simulink model "bibli_SM_QUEVAL_20240121_R2021a"  (Simulink 9.3)
settings: Solver=VariableStepAuto  StartTime=0.0  StopTime=10  MaxStep=1e-3  RelTol=1e-3
values from neighbouring files (symbols this model uses):
  Fif = 0.259*3    (= 0.777)    [param_PMSM.m]
  J = 0.5    [param_EESM.m]    (also in param_EESMdampers.m; param_PMSM.m)
  Ld = 1.59e-2    (= 0.0159)    [param_EESM.m]    (also in param_EESMdampers.m; param_PMSM.m)
  Lq = 1.59e-2    (= 0.0159)    [param_EESM.m]    (also in param_EESMdampers.m; param_PMSM.m)
  npp = 2    [param_EESM.m]    (also in param_EESMdampers.m; param_PMSM.m)
undefined symbols (not defined in the file or in its folder): iao_pd_si, ibo_pd_si, ico_pd_si, Ts
undefined symbols (not defined in the file): Clark, fd, InvClark, INVL, M, R
libraries: powerlib x42
(part 1 of 2)
settings Model: Creator=Loïc Queval  LastModifiedBy=Loïc Queval
settings DataIOCC: SaveFormat=Dataset  SignalLoggingSaveFormat=Dataset  ReturnWorkspaceOutputs=on
settings OptimizationCC: LifeSpan=auto
settings DebuggingCC: UnderspecifiedInitializationDetection=Simplified  MergeDetectMultiDrivingBlocksExec=error  FcnCallInpInsideContextMsg=error  UnconnectedInputMsg=none  UnconnectedOutputMsg=none  UnconnectedLineMsg=none  SFUnexpectedBacktrackingDiag=error  SFNoUnconditionalDefaultTransitionDiag=error  SFExecutionAtInitializationDiag=warning  ArithmeticOperatorsInVariantConditions=error
settings HardwareCC: ProdBitPerPointer=64  ProdBitPerSizeT=64  ProdBitPerPtrDiffT=64  ProdLargestAtomicFloat=Float  ProdIntDivRoundTo=Zero  ProdEndianess=LittleEndian  ProdWordSize=64  ProdHWDeviceType=Intel->x86-64 (Windows64)
settings ModelReferenceCC: EnableRefExpFcnMdlSchedulingChecks=off  PropagateSignalLabelsOutOfModel=on
settings SFSimCC: SimUseLocalCustomCode=on
settings RTWCC: RTWUseLocalCustomCode=on
settings CodeAppCC: StateflowObjectComments=off
settings GRTTargetCC: TargetLangStandard=C99 (ISO)  CombineOutputUpdateFcns=on  GRTInterface=off
settings ConfigComp: CovMetricSettings=dwe  CovSaveCumulativeToWorkspaceVar=off  CovSaveSingleToWorkspaceVar=off  CovExternalEMLEnable=on

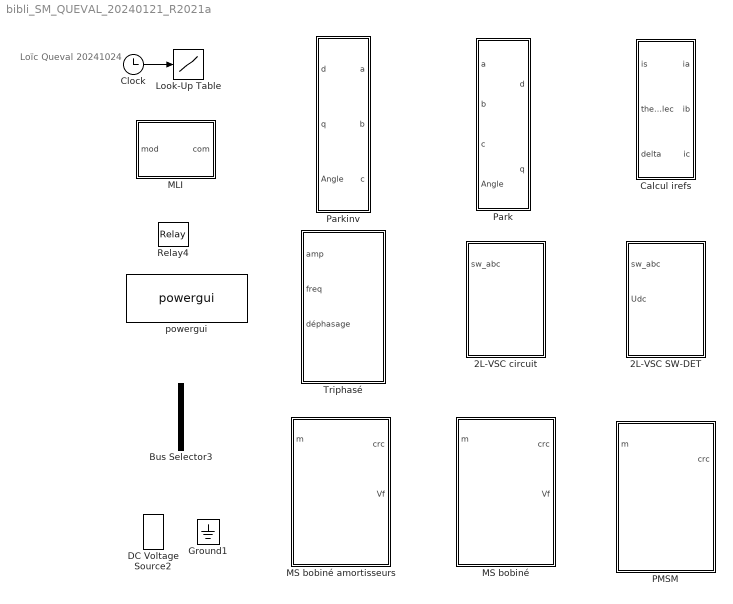
== system bibli_SM_QUEVAL_20240121_R2021a ==
  note: Loïc Queval
      | 20241024
  2L-VSC SW-DET : Subsystem
  2L-VSC circuit : Subsystem
  Bus Selector3 : BusSelector  OutputSignals=Cm,Vit,ia,v_an
  Calcul irefs : Subsystem
  Clock : Clock
  DC Voltage Source2 : powerlib/Electrical Sources/DC Voltage Source  Amplitude=300  Measurements=None
  Ground1 : powerlib/Elements/Ground  LConnTagsString=a
  Look-Up Table : Lookup  InputValues=[0 4 4 6 6 10]  Table=[0 0 30 30 100 100]  SaturateOnIntegerOverflow=on
  MLI : Subsystem
  MS bobiné : Subsystem
  MS bobiné amortisseurs : Subsystem
  PMSM : Subsystem
  Park : Subsystem
  Parkinv : Subsystem
  Relay4 : Relay  OnSwitchValue=1  OffSwitchValue=-1
  Triphasé : Subsystem
  powergui : powerlib/powergui  SimulationMode=Continuous  SampleTime=Ts  frequency=60  Iterations=50  frequencyindice=0  Pbase=100e6  ErrMax=1e-4  UnitsV=kV  UnitsW=MW  buscounter=0  FunctionMessages=off  echomessages=off  EnableUseOfTLC=off  CurrentSourceSwitches=off  DisableSnubberDevices=off  DisableRonSwitches=off  DisableVfSwitches=off  DisplayEquations=off  AutomaticDiscreteSolvers=off  SolverType=Tustin/Backward Euler (TBE)  Interpol=off  ExternalGateDelay=off  methode=off  Ts=0  x0status=blocks  SPID=off  SwTol=0  HookPort=off  NonlinearTolerance=1e-4  nMaxIteration=100  ContinueOnMaxIteration=off  RestoreLinks=warning  ResistiveCurrentMeasurement=off  Frange=[0:2:500]  Ylog=off  Xlog=on  ShowGrid=off  save=off  variable=ZData  structure=data_PWM  ZoomFFT=off  StartTime=0.02  cycles=1  DisplayStyle=1  fundamental=50  FreqAxis=on  MaxFrequency=1000  frequencyindicesteady=1  RmsSteady=1  display=off
  wires:
  Clock/1 -> Look-Up Table/1

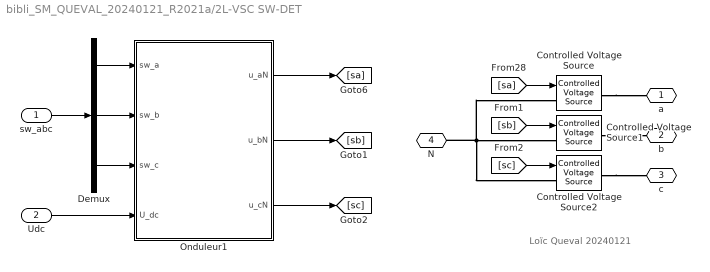
== system bibli_SM_QUEVAL_20240121_R2021a/2L-VSC SW-DET ==
  note: Loïc Queval
      | 20240121
  sw_abc : Inport
  Udc : Inport  Port=2
  Controlled Voltage Source : powerlib/Electrical Sources/Controlled Voltage Source  Initialize=off  Source_Type=AC  Amplitude=0  Phase=0  Frequency=0  Measurements=None
  Controlled Voltage Source1 : powerlib/Electrical Sources/Controlled Voltage Source  Initialize=off  Source_Type=AC  Amplitude=0  Phase=0  Frequency=0  Measurements=None
  Controlled Voltage Source2 : powerlib/Electrical Sources/Controlled Voltage Source  Initialize=off  Source_Type=AC  Amplitude=0  Phase=0  Frequency=0  Measurements=None
  Demux : Demux  Outputs=3
  Onduleur1 : Subsystem
  a : PMIOPort  Side=Right
  b : PMIOPort  Port=2  Side=Right
  c : PMIOPort  Port=3  Side=Right
  N : PMIOPort  Port=4  Side=Left
  wires:
  Demux/1 -> Onduleur1/1(sw_a)
  [sa] -> Controlled Voltage Source/1
  [sb] -> Controlled Voltage Source1/1
  [sc] -> Controlled Voltage Source2/1
  Demux/2 -> Onduleur1/2(sw_b)
  Demux/3 -> Onduleur1/3(sw_c)
  Udc/1 -> Onduleur1/4(U_dc)
  Onduleur1/3(u_cN) -> [sc]
  Onduleur1/1(u_aN) -> [sa]
  Onduleur1/2(u_bN) -> [sb]
  sw_abc/1 -> Demux/1
  connections:
  Controlled Voltage Source/RConn1 -- a/RConn1
  Controlled Voltage Source1/RConn1 -- b/RConn1
  Controlled Voltage Source2/RConn1 -- c/RConn1
  N/RConn1 -- Controlled Voltage Source2/LConn1 -- Controlled Voltage Source1/LConn1 -- Controlled Voltage Source/LConn1

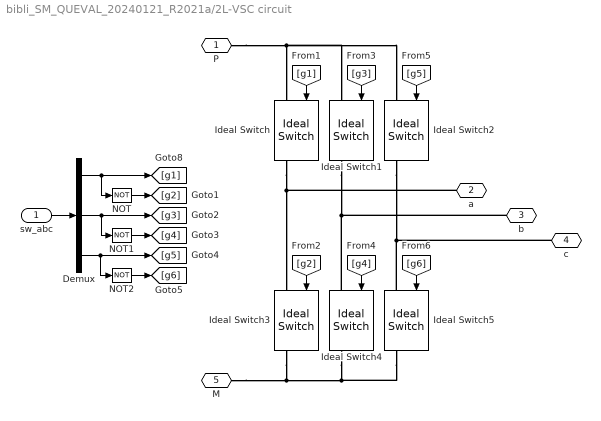
== system bibli_SM_QUEVAL_20240121_R2021a/2L-VSC circuit ==
  sw_abc : Inport
  Demux : Demux  Outputs=3
  Ideal Switch{,1..5} (6 alike) : powerlib/Power Electronics/Ideal Switch  Ron=0.001  Lon=0  IC=0  Rs=1e5  Cs=inf  Measurements=on
  NOT : Logic  Operator=NOT  IconShape=distinctive  AllPortsSameDT=off  OutDataTypeStr=boolean
  NOT1 : Logic  Operator=NOT  IconShape=distinctive  AllPortsSameDT=off  OutDataTypeStr=boolean
  NOT2 : Logic  Operator=NOT  IconShape=distinctive  AllPortsSameDT=off  OutDataTypeStr=boolean
  P : PMIOPort  Side=Left
  a : PMIOPort  Port=2  Side=Right
  b : PMIOPort  Port=3  Side=Right
  c : PMIOPort  Port=4  Side=Right
  M : PMIOPort  Port=5  Side=Left
  wires:
  sw_abc/1 -> Demux/1
  [g1] -> Ideal Switch/1
  [g2] -> Ideal Switch3/1
  [g3] -> Ideal Switch1/1
  [g4] -> Ideal Switch4/1
  [g5] -> Ideal Switch2/1
  [g6] -> Ideal Switch5/1
  NOT1/1 -> [g4]
  Demux/1 -> NOT/1, [g1]
  NOT/1 -> [g2]
  NOT2/1 -> [g6]
  Demux/2 -> NOT1/1, [g3]
  Demux/3 -> NOT2/1, [g5]
  connections:
  b/RConn1 -- Ideal Switch4/LConn1 -- Ideal Switch1/RConn1
  a/RConn1 -- Ideal Switch/RConn1 -- Ideal Switch3/LConn1
  M/RConn1 -- Ideal Switch3/RConn1 -- Ideal Switch5/RConn1 -- Ideal Switch4/RConn1
  P/RConn1 -- Ideal Switch2/LConn1 -- Ideal Switch1/LConn1 -- Ideal Switch/LConn1
  c/RConn1 -- Ideal Switch5/LConn1 -- Ideal Switch2/RConn1

== system bibli_SM_QUEVAL_20240121_R2021a/Calcul irefs ==
  is : Inport
  thetelec : Inport  Port=2
  delta : Inport  Port=3
  Fcn : Fcn  Expr=u[1]*cos(u[2]+u[3])
  Fcn1 : Fcn  Expr=u[1]*cos(u[2]-2*pi/3+u[3])
  Fcn2 : Fcn  Expr=u[1]*cos(u[2]-4*pi/3+u[3])
  Mux : Mux  Inputs=3
  ia : Outport  InitialOutput=0  VectorParamsAs1DForOutWhenUnconnected=off
  ib : Outport  Port=2  InitialOutput=0  VectorParamsAs1DForOutWhenUnconnected=off
  ic : Outport  Port=3  InitialOutput=0  VectorParamsAs1DForOutWhenUnconnected=off
  wires:
  Mux/1 -> Fcn1/1, Fcn2/1, Fcn/1
  Fcn/1 -> ia/1
  is/1 -> Mux/1
  Fcn1/1 -> ib/1
  thetelec/1 -> Mux/2
  Fcn2/1 -> ic/1
  delta/1 -> Mux/3

== system bibli_SM_QUEVAL_20240121_R2021a/MLI ==
  note: Définir la fréquence de découpage fd
  mod : Inport
  Relay : Relay  OnSwitchValue=0  OffSwitchValue=0
  Repeating Sequence : Subsystem  mask(Repeating table){Parameter1=[0 0.25/fd 0.75/fd 1/fd], Parameter2=[0 1 -1 0]}
      mask prompts: Parameter1 "Time values:"; Parameter2 "Output values:"
      mask help:
      | Repeating table.
      | Enter values of time and output for first cycle.
      mask init:
      | period = max(@1); t = @1; y = @2;
      mask Help: Repeats cycle given in table. Time values should be monotonically increasing.
      mask Display: plot([t,t+period,t+2*period],[y,y,y])
  Sum : Sum  Inputs=+-  InputSameDT=on  SaturateOnIntegerOverflow=on  OutDataTypeStr=Inherit: Same as first input
  com : Outport  VectorParamsAs1DForOutWhenUnconnected=off
  wires:
  Repeating Sequence/1(out_1) -> Sum/2
  Sum/1 -> Relay/1
  mod/1 -> Sum/1
  Relay/1 -> com/1

== system bibli_SM_QUEVAL_20240121_R2021a/MS bobiné ==
  note: ELECTRICAL TERMINATORS
      | OF THE MACHINE
  note: <----- ia
  note: Loïc Queval
      | 20240109
  note: current must go out!
  crc : Inport
  Vf : Inport  Port=2
  CURRENT INJECTION SYSTEM Converts Simulink signals into currents : Subsystem
  Gain : Gain  Gain=-1
  MS bobiné : Subsystem
  VOLTAGE MEASUREMENT SYSTEM Converts voltages into  Simulink signals : Subsystem
  n : PMIOPort  Side=Left
  a : PMIOPort  Port=2  Side=Right
  b : PMIOPort  Port=3  Side=Right
  c : PMIOPort  Port=4  Side=Right
  m : Outport
  wires:
  VOLTAGE MEASUREMENT SYSTEM Converts voltages into  Simulink signals/1(voltages) -> MS bobiné/1(voltages)
  MS bobiné/1(currents) -> Gain/1
  MS bobiné/2(m) -> m/1
  Gain/1 -> CURRENT INJECTION SYSTEM Converts Simulink signals into currents/1(currents)
  Vf/1 -> MS bobiné/3(Vf)
  crc/1 -> MS bobiné/2(crc)
  connections:
  a/RConn1 -- CURRENT INJECTION SYSTEM Converts Simulink signals into currents/RConn1 -- VOLTAGE MEASUREMENT SYSTEM Converts voltages into  Simulink signals/LConn1
  VOLTAGE MEASUREMENT SYSTEM Converts voltages into  Simulink signals/LConn2 -- CURRENT INJECTION SYSTEM Converts Simulink signals into currents/RConn2 -- b/RConn1
  VOLTAGE MEASUREMENT SYSTEM Converts voltages into  Simulink signals/LConn3 -- CURRENT INJECTION SYSTEM Converts Simulink signals into currents/RConn3 -- c/RConn1
  n/RConn1 -- CURRENT INJECTION SYSTEM Converts Simulink signals into currents/RConn4 -- VOLTAGE MEASUREMENT SYSTEM Converts voltages into  Simulink signals/LConn4

== system bibli_SM_QUEVAL_20240121_R2021a/MS bobiné amortisseurs ==
  note: ELECTRICAL TERMINATORS
      | OF THE MACHINE
  note: <----- ia
  note: Loïc Queval
      | 20240109
  note: current must go out!
  crc : Inport
  Vf : Inport  Port=2
  CURRENT INJECTION SYSTEM Converts Simulink signals into currents : Subsystem
  Gain : Gain  Gain=-1
  MS bobiné amortisseurs : Subsystem
  VOLTAGE MEASUREMENT SYSTEM Converts voltages into  Simulink signals : Subsystem
  n : PMIOPort  Side=Left
  a : PMIOPort  Port=2  Side=Right
  b : PMIOPort  Port=3  Side=Right
  c : PMIOPort  Port=4  Side=Right
  m : Outport
  wires:
  VOLTAGE MEASUREMENT SYSTEM Converts voltages into  Simulink signals/1(voltages) -> MS bobiné amortisseurs/1(voltages)
  MS bobiné amortisseurs/1(currents) -> Gain/1
  MS bobiné amortisseurs/2(m) -> m/1
  Gain/1 -> CURRENT INJECTION SYSTEM Converts Simulink signals into currents/1(currents)
  crc/1 -> MS bobiné amortisseurs/2(crc)
  Vf/1 -> MS bobiné amortisseurs/3(Vf)
  connections:
  a/RConn1 -- CURRENT INJECTION SYSTEM Converts Simulink signals into currents/RConn1 -- VOLTAGE MEASUREMENT SYSTEM Converts voltages into  Simulink signals/LConn1
  VOLTAGE MEASUREMENT SYSTEM Converts voltages into  Simulink signals/LConn2 -- CURRENT INJECTION SYSTEM Converts Simulink signals into currents/RConn2 -- b/RConn1
  VOLTAGE MEASUREMENT SYSTEM Converts voltages into  Simulink signals/LConn3 -- CURRENT INJECTION SYSTEM Converts Simulink signals into currents/RConn3 -- c/RConn1
  n/RConn1 -- CURRENT INJECTION SYSTEM Converts Simulink signals into currents/RConn4 -- VOLTAGE MEASUREMENT SYSTEM Converts voltages into  Simulink signals/LConn4

== system bibli_SM_QUEVAL_20240121_R2021a/PMSM ==
  note: ELECTRICAL TERMINATORS
      | OF THE MACHINE
  note: <----- ia
  note: Loïc Queval
      | 20240120
  note: current must go out!
  crc : Inport
  CURRENT INJECTION SYSTEM Converts Simulink signals into currents : Subsystem
  Gain : Gain  Gain=-1
  PMSM : Subsystem
  VOLTAGE MEASUREMENT SYSTEM Converts voltages into  Simulink signals : Subsystem
  n : PMIOPort  Side=Left
  a : PMIOPort  Port=2  Side=Right
  b : PMIOPort  Port=3  Side=Right
  c : PMIOPort  Port=4  Side=Right
  m : Outport
  wires:
  VOLTAGE MEASUREMENT SYSTEM Converts voltages into  Simulink signals/1(voltages) -> PMSM/1(voltages)
  PMSM/1(currents) -> Gain/1
  PMSM/2(m) -> m/1
  Gain/1 -> CURRENT INJECTION SYSTEM Converts Simulink signals into currents/1(currents)
  crc/1 -> PMSM/2(crc)
  connections:
  CURRENT INJECTION SYSTEM Converts Simulink signals into currents/RConn1 -- a/RConn1 -- VOLTAGE MEASUREMENT SYSTEM Converts voltages into  Simulink signals/LConn1
  CURRENT INJECTION SYSTEM Converts Simulink signals into currents/RConn2 -- VOLTAGE MEASUREMENT SYSTEM Converts voltages into  Simulink signals/LConn2 -- b/RConn1
  VOLTAGE MEASUREMENT SYSTEM Converts voltages into  Simulink signals/LConn3 -- c/RConn1 -- CURRENT INJECTION SYSTEM Converts Simulink signals into currents/RConn3
  n/RConn1 -- CURRENT INJECTION SYSTEM Converts Simulink signals into currents/RConn4 -- VOLTAGE MEASUREMENT SYSTEM Converts voltages into  Simulink signals/LConn4

== system bibli_SM_QUEVAL_20240121_R2021a/Park ==
  a : Inport
  b : Inport  Port=2
  c : Inport  Port=3
  Angle : Inport  Port=4
  Clark : Subsystem
  Rotation : Subsystem
  Trigonometric Function : Trigonometry
  Trigonometric Function1 : Trigonometry  Operator=cos
  d : Outport  InitialOutput=0  VectorParamsAs1DForOutWhenUnconnected=off
  q : Outport  Port=2  InitialOutput=0  VectorParamsAs1DForOutWhenUnconnected=off
  wires:
  Rotation/1(d) -> d/1
  Rotation/2(q) -> q/1
  b/1 -> Clark/2(b)
  c/1 -> Clark/3(c)
  a/1 -> Clark/1(a)
  Clark/1(alpha) -> Rotation/3(alpha)
  Clark/2(beta) -> Rotation/4(beta)
  Trigonometric Function/1 -> Rotation/2(sin)
  Trigonometric Function1/1 -> Rotation/1(cos)
  Angle/1 -> Trigonometric Function1/1, Trigonometric Function/1

== system bibli_SM_QUEVAL_20240121_R2021a/Parkinv ==
  d : Inport
  q : Inport  Port=2
  Angle : Inport  Port=3
  ClarkInv : Subsystem
  Rotation Inverse : Subsystem
  Trigonometric Function : Trigonometry
  Trigonometric Function1 : Trigonometry  Operator=cos
  a : Outport  InitialOutput=0  VectorParamsAs1DForOutWhenUnconnected=off
  b : Outport  Port=2  InitialOutput=0  VectorParamsAs1DForOutWhenUnconnected=off
  c : Outport  Port=3  InitialOutput=0  VectorParamsAs1DForOutWhenUnconnected=off
  wires:
  Rotation Inverse/1(alpha) -> ClarkInv/1(alpha)
  ClarkInv/1(a) -> a/1
  ClarkInv/2(b) -> b/1
  d/1 -> Rotation Inverse/3(d)
  ClarkInv/3(c) -> c/1
  q/1 -> Rotation Inverse/4(q)
  Rotation Inverse/2(beta) -> ClarkInv/2(beta)
  Trigonometric Function/1 -> Rotation Inverse/2(sin)
  Trigonometric Function1/1 -> Rotation Inverse/1(cos)
  Angle/1 -> Trigonometric Function1/1, Trigonometric Function/1

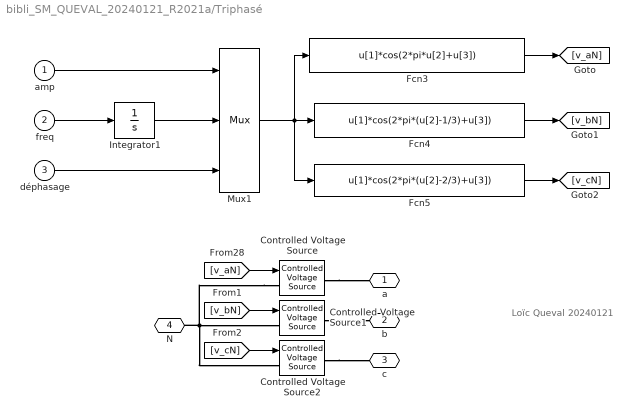
== system bibli_SM_QUEVAL_20240121_R2021a/Triphasé ==
  note: Loïc Queval
      | 20240121
  amp : Inport
  freq : Inport  Port=2
  déphasage : Inport  Port=3
  Controlled Voltage Source : powerlib/Electrical Sources/Controlled Voltage Source  Initialize=on  Source_Type=AC  Amplitude=0  Phase=0  Frequency=0  Measurements=None
  Controlled Voltage Source1 : powerlib/Electrical Sources/Controlled Voltage Source  Initialize=on  Source_Type=AC  Amplitude=0  Phase=0  Frequency=0  Measurements=None
  Controlled Voltage Source2 : powerlib/Electrical Sources/Controlled Voltage Source  Initialize=on  Source_Type=AC  Amplitude=0  Phase=0  Frequency=0  Measurements=None
  Fcn3 : Fcn  Expr=u[1]*cos(2*pi*u[2]+u[3])
  Fcn4 : Fcn  Expr=u[1]*cos(2*pi*(u[2]-1/3)+u[3])
  Fcn5 : Fcn  Expr=u[1]*cos(2*pi*(u[2]-2/3)+u[3])
  Integrator1 : Integrator
  Mux1 : Mux  Inputs=3
  a : PMIOPort  Side=Right
  b : PMIOPort  Port=2  Side=Right
  c : PMIOPort  Port=3  Side=Right
  N : PMIOPort  Port=4  Side=Left
  wires:
  Fcn5/1 -> [v_cN]
  Fcn4/1 -> [v_bN]
  Fcn3/1 -> [v_aN]
  [v_aN] -> Controlled Voltage Source/1
  [v_bN] -> Controlled Voltage Source1/1
  [v_cN] -> Controlled Voltage Source2/1
  Integrator1/1 -> Mux1/2
  amp/1 -> Mux1/1
  Mux1/1 -> Fcn4/1, Fcn5/1, Fcn3/1
  freq/1 -> Integrator1/1
  déphasage/1 -> Mux1/3
  connections:
  Controlled Voltage Source/LConn1 -- N/RConn1 -- Controlled Voltage Source2/LConn1 -- Controlled Voltage Source1/LConn1
  Controlled Voltage Source1/RConn1 -- b/RConn1
  Controlled Voltage Source2/RConn1 -- c/RConn1
  Controlled Voltage Source/RConn1 -- a/RConn1

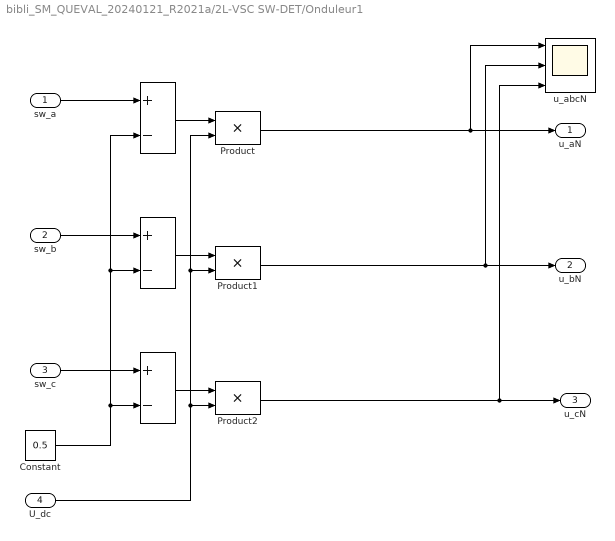
== system bibli_SM_QUEVAL_20240121_R2021a/2L-VSC SW-DET/Onduleur1 ==
  sw_a : Inport
  sw_b : Inport  Port=2
  sw_c : Inport  Port=3
  U_dc : Inport  Port=4
  " " : Sum  Inputs=+-  InputSameDT=on  SaturateOnIntegerOverflow=on  OutDataTypeStr=Inherit: Same as first input
  "  " : Sum  Inputs=+-  InputSameDT=on  SaturateOnIntegerOverflow=on  OutDataTypeStr=Inherit: Same as first input
  "   " : Sum  Inputs=+-  InputSameDT=on  SaturateOnIntegerOverflow=on  OutDataTypeStr=Inherit: Same as first input
  Constant : Constant  Value=0.5
  Product : Product  InputSameDT=on  SaturateOnIntegerOverflow=on  OutDataTypeStr=Inherit: Same as first input
  Product1 : Product  InputSameDT=on  SaturateOnIntegerOverflow=on  OutDataTypeStr=Inherit: Same as first input
  Product2 : Product  InputSameDT=on  SaturateOnIntegerOverflow=on  OutDataTypeStr=Inherit: Same as first input
  u_abcN : Scope  NumInputPorts=3
  u_aN : Outport  VectorParamsAs1DForOutWhenUnconnected=off
  u_bN : Outport  Port=2  VectorParamsAs1DForOutWhenUnconnected=off
  u_cN : Outport  Port=3  VectorParamsAs1DForOutWhenUnconnected=off
  wires:
  sw_a/1 -> " "/1
  sw_b/1 -> "   "/1
  sw_c/1 -> "  "/1
  Product/1 -> u_abcN/1, u_aN/1
  " "/1 -> Product/1
  "   "/1 -> Product1/1
  "  "/1 -> Product2/1
  U_dc/1 -> Product/2, Product1/2, Product2/2
  Constant/1 -> " "/2, "   "/2, "  "/2
  Product1/1 -> u_abcN/2, u_bN/1
  Product2/1 -> u_abcN/3, u_cN/1

== system bibli_SM_QUEVAL_20240121_R2021a/MLI/Repeating Sequence ==
  Clock : Clock
  Fcn1 : Fcn  Expr=rem(u[1],period)
  Look-Up Table : Lookup  InputValues=t  Table=y  SaturateOnIntegerOverflow=on
  out_1 : Outport  InitialOutput=0  VectorParamsAs1DForOutWhenUnconnected=off
  wires:
  Look-Up Table/1 -> out_1/1
  Clock/1 -> Fcn1/1
  Fcn1/1 -> Look-Up Table/1

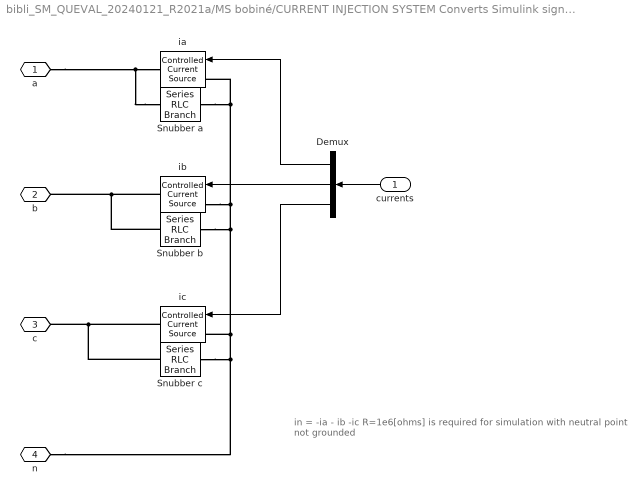
== system bibli_SM_QUEVAL_20240121_R2021a/MS bobiné/CURRENT INJECTION SYSTEM Converts Simulink signals into currents ==
  note: in = -ia - ib -ic
      | R=1e6[ohms] is required for simulation with neutral point not grounded
  currents : Inport
  Demux : Demux  Outputs=3
  Snubber a : powerlib/Elements/Series RLC Branch  LConnTagsString=__new0  RConnTagsString=__new0  BranchType=R  Resistance=1e6  Inductance=1e-3  SetiL0=off  InitialCurrent=0  Capacitance=1e-6  Setx0=off  InitialVoltage=0  Measurements=None
  Snubber b : powerlib/Elements/Series RLC Branch  LConnTagsString=__new0  RConnTagsString=__new0  BranchType=R  Resistance=1e6  Inductance=1e-3  SetiL0=off  InitialCurrent=0  Capacitance=1e-6  Setx0=off  InitialVoltage=0  Measurements=None
  Snubber c : powerlib/Elements/Series RLC Branch  LConnTagsString=__new0  RConnTagsString=__new0  BranchType=R  Resistance=1e6  Inductance=1e-3  SetiL0=off  InitialCurrent=0  Capacitance=1e-6  Setx0=off  InitialVoltage=0  Measurements=None
  ia : powerlib/Electrical Sources/Controlled Current Source  Initialize=off  Source_Type=DC  Amplitude=-iao_pd_si  Phase=0  Frequency=0  Measurements=None
  ib : powerlib/Electrical Sources/Controlled Current Source  Initialize=off  Source_Type=DC  Amplitude=-ibo_pd_si  Phase=0  Frequency=0  Measurements=None
  ic : powerlib/Electrical Sources/Controlled Current Source  Initialize=off  Source_Type=DC  Amplitude=-ico_pd_si  Phase=0  Frequency=0  Measurements=None
  a : PMIOPort  Side=Right
  b : PMIOPort  Port=2  Side=Right
  c : PMIOPort  Port=3  Side=Right
  n : PMIOPort  Port=4  Side=Right
  wires:
  Demux/1 -> ia/1
  Demux/2 -> ib/1
  currents/1 -> Demux/1
  Demux/3 -> ic/1
  connections:
  Snubber a/LConn1 -- a/RConn1 -- ia/RConn1
  ib/RConn1 -- b/RConn1 -- Snubber b/LConn1
  Snubber b/RConn1 -- Snubber a/RConn1 -- ia/LConn1 -- ib/LConn1 -- ic/LConn1 -- Snubber c/RConn1 -- n/RConn1
  Snubber c/LConn1 -- ic/RConn1 -- c/RConn1

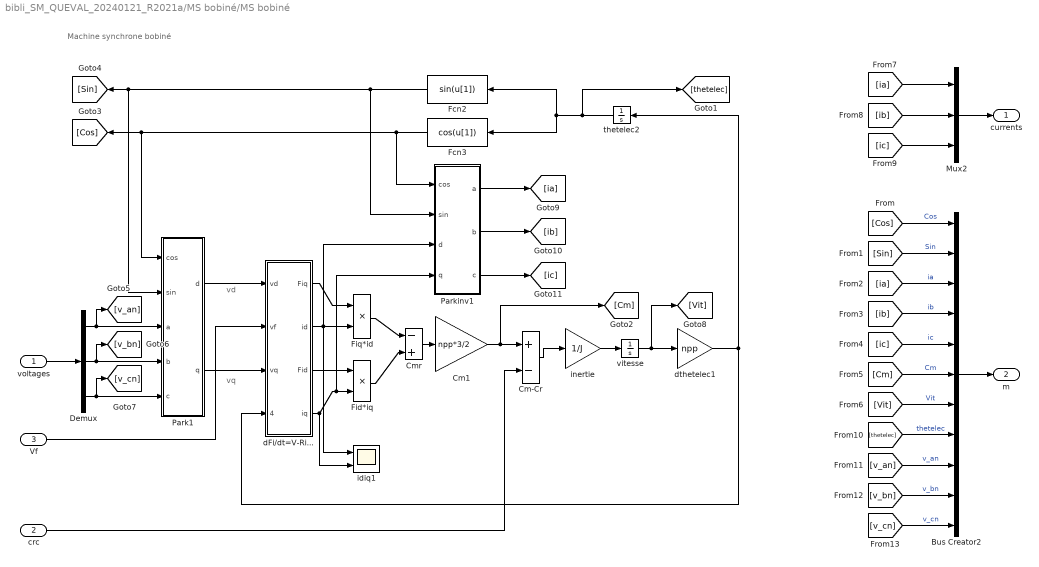
== system bibli_SM_QUEVAL_20240121_R2021a/MS bobiné/MS bobiné ==
  note: Machine synchrone bobiné
  note: vd
  note: vq
  voltages : Inport
  crc : Inport  Port=2
  Vf : Inport  Port=3
  Bus Creator2 : BusCreator  Inputs=11
  Cm-Cr : Sum  Inputs=+-  InputSameDT=on  SaturateOnIntegerOverflow=on  OutDataTypeStr=Inherit: Same as first input
  Cm1 : Gain  Gain=npp*3/2  SaturateOnIntegerOverflow=on  OutDataTypeStr=Inherit: Same as input  ParamDataTypeStr=Inherit: Same as input
  Cmr : Sum  Inputs=-+  InputSameDT=on  SaturateOnIntegerOverflow=on  OutDataTypeStr=Inherit: Same as first input
  Demux : Demux  Outputs=3
  Fcn2 : Fcn
  Fcn3 : Fcn  Expr=cos(u[1])
  "Fid*iq " : Product  InputSameDT=on  RndMeth=Zero  SaturateOnIntegerOverflow=on  OutDataTypeStr=Inherit: Same as first input
  Fiq*id : Product  InputSameDT=on  RndMeth=Zero  SaturateOnIntegerOverflow=on  OutDataTypeStr=Inherit: Same as first input
  Mux2 : Mux  Inputs=3
  Park1 : Subsystem
  Parkinv1 : Subsystem
  dFi/dt=V-Ri... : Subsystem
  dthetelec1 : Gain  Gain=npp  SaturateOnIntegerOverflow=on  OutDataTypeStr=Inherit: Same as input  ParamDataTypeStr=Inherit: Same as input
  idiq1 : Scope  NumInputPorts=2
  inertie : Gain  Gain=1/J  SaturateOnIntegerOverflow=on  OutDataTypeStr=Inherit: Same as input  ParamDataTypeStr=Inherit: Same as input
  thetelec2 : Integrator
  vitesse : Integrator
  currents : Outport
  m : Outport  Port=2
  wires:
  Mux2/1 -> currents/1
  Bus Creator2/1 -> m/1
  [Vit] -> Bus Creator2/7  "Vit"
  [Cm] -> Bus Creator2/6  "Cm"
  [ic] -> Bus Creator2/5  "ic"
  [ib] -> Bus Creator2/4  "ib"
  [ia] -> Bus Creator2/3  "ia"
  [Sin] -> Bus Creator2/2  "Sin"
  [Cos] -> Bus Creator2/1  "Cos"
  [ia] -> Mux2/1
  [ib] -> Mux2/2
  [ic] -> Mux2/3
  [thetelec] -> Bus Creator2/8  "thetelec"
  dFi/dt=V-Ri.../3(Fid) -> "Fid*iq "/1
  "Fid*iq "/1 -> Cmr/2
  Fiq*id/1 -> Cmr/1
  Fcn3/1 -> Parkinv1/1(cos), Park1/1(cos), [Cos]
  dFi/dt=V-Ri.../1(Fiq) -> Fiq*id/1
  Demux/2 -> [v_bn], Park1/4(b)
  Cmr/1 -> Cm1/1
  dFi/dt=V-Ri.../4(iq) -> idiq1/2, Parkinv1/4(q), "Fid*iq "/2
  Park1/1(d) -> dFi/dt=V-Ri.../1(vd)
  dFi/dt=V-Ri.../2(id) -> idiq1/1, Parkinv1/3(d), Fiq*id/2
  Cm-Cr/1 -> inertie/1
  Vf/1 -> dFi/dt=V-Ri.../2(vf)
  vitesse/1 -> [Vit], dthetelec1/1
  Fcn2/1 -> Parkinv1/2(sin), [Sin], Park1/2(sin)
  inertie/1 -> vitesse/1
  thetelec2/1 -> [thetelec], Fcn2/1, Fcn3/1
  Demux/3 -> [v_cn], Park1/5(c)
  Cm1/1 -> [Cm], Cm-Cr/1
  dthetelec1/1 -> thetelec2/1, dFi/dt=V-Ri.../4(dthetelec)
  Parkinv1/1(a) -> [ia]
  Parkinv1/3(c) -> [ic]
  Demux/1 -> [v_an], Park1/3(a)
  Parkinv1/2(b) -> [ib]
  Park1/2(q) -> dFi/dt=V-Ri.../3(vq)
  voltages/1 -> Demux/1
  crc/1 -> Cm-Cr/2
  [v_cn] -> Bus Creator2/11  "v_cn"
  [v_bn] -> Bus Creator2/10  "v_bn"
  [v_an] -> Bus Creator2/9  "v_an"

== system bibli_SM_QUEVAL_20240121_R2021a/MS bobiné/VOLTAGE MEASUREMENT SYSTEM Converts voltages into  Simulink signals ==
  Mux : Mux  Inputs=3
  v_an : powerlib/Measurements/Voltage Measurement  PhasorSimulation=off  OutputType=Complex  PSBequivalent=0
  v_bn : powerlib/Measurements/Voltage Measurement  PhasorSimulation=off  OutputType=Complex  PSBequivalent=0
  v_cn : powerlib/Measurements/Voltage Measurement  PhasorSimulation=off  OutputType=Complex  PSBequivalent=0
  a : PMIOPort  Side=Left
  b : PMIOPort  Port=2  Side=Left
  c : PMIOPort  Port=3  Side=Left
  n : PMIOPort  Port=4  Side=Left
  voltages : Outport
  wires:
  v_an/1 -> Mux/1
  v_bn/1 -> Mux/2
  Mux/1 -> voltages/1
  v_cn/1 -> Mux/3
  connections:
  v_an/LConn1 -- a/RConn1
  b/RConn1 -- v_bn/LConn1
  c/RConn1 -- v_cn/LConn1
  n/RConn1 -- v_bn/LConn2 -- v_an/LConn2 -- v_cn/LConn2

== system bibli_SM_QUEVAL_20240121_R2021a/MS bobiné amortisseurs/CURRENT INJECTION SYSTEM Converts Simulink signals into currents ==
  note: in = -ia - ib -ic
      | R=1e6[ohms] is required for simulation with neutral point not grounded
  currents : Inport
  Demux : Demux  Outputs=3
  Snubber a : powerlib/Elements/Series RLC Branch  LConnTagsString=__new0  RConnTagsString=__new0  BranchType=R  Resistance=1e6  Inductance=1e-3  SetiL0=off  InitialCurrent=0  Capacitance=1e-6  Setx0=off  InitialVoltage=0  Measurements=None
  Snubber b : powerlib/Elements/Series RLC Branch  LConnTagsString=__new0  RConnTagsString=__new0  BranchType=R  Resistance=1e6  Inductance=1e-3  SetiL0=off  InitialCurrent=0  Capacitance=1e-6  Setx0=off  InitialVoltage=0  Measurements=None
  Snubber c : powerlib/Elements/Series RLC Branch  LConnTagsString=__new0  RConnTagsString=__new0  BranchType=R  Resistance=1e6  Inductance=1e-3  SetiL0=off  InitialCurrent=0  Capacitance=1e-6  Setx0=off  InitialVoltage=0  Measurements=None
  ia : powerlib/Electrical Sources/Controlled Current Source  Initialize=off  Source_Type=DC  Amplitude=-iao_pd_si  Phase=0  Frequency=0  Measurements=None
  ib : powerlib/Electrical Sources/Controlled Current Source  Initialize=off  Source_Type=DC  Amplitude=-ibo_pd_si  Phase=0  Frequency=0  Measurements=None
  ic : powerlib/Electrical Sources/Controlled Current Source  Initialize=off  Source_Type=DC  Amplitude=-ico_pd_si  Phase=0  Frequency=0  Measurements=None
  a : PMIOPort  Side=Right
  b : PMIOPort  Port=2  Side=Right
  c : PMIOPort  Port=3  Side=Right
  n : PMIOPort  Port=4  Side=Right
  wires:
  Demux/1 -> ia/1
  Demux/2 -> ib/1
  currents/1 -> Demux/1
  Demux/3 -> ic/1
  connections:
  Snubber a/LConn1 -- a/RConn1 -- ia/RConn1
  ib/RConn1 -- b/RConn1 -- Snubber b/LConn1
  Snubber b/RConn1 -- Snubber a/RConn1 -- ia/LConn1 -- ib/LConn1 -- ic/LConn1 -- Snubber c/RConn1 -- n/RConn1
  Snubber c/LConn1 -- ic/RConn1 -- c/RConn1

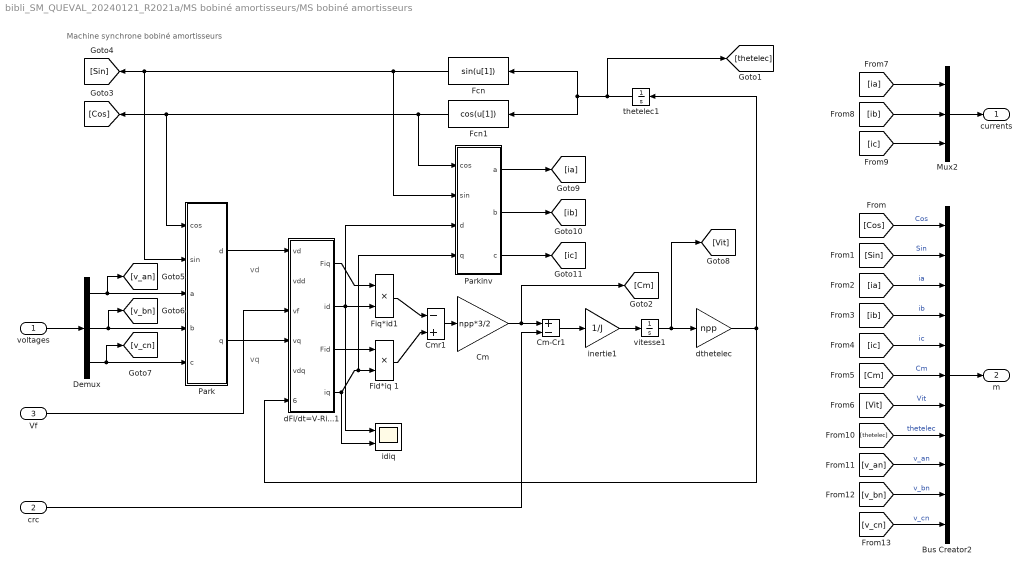
== system bibli_SM_QUEVAL_20240121_R2021a/MS bobiné amortisseurs/MS bobiné amortisseurs ==
  note: Machine synchrone bobiné amortisseurs
  note: vq
  note: vd
  voltages : Inport
  crc : Inport  Port=2
  Vf : Inport  Port=3
  Bus Creator2 : BusCreator  Inputs=11
  Cm : Gain  Gain=npp*3/2  SaturateOnIntegerOverflow=on  OutDataTypeStr=Inherit: Same as input  ParamDataTypeStr=Inherit: Same as input
  Cm-Cr1 : Sum  Inputs=+-  InputSameDT=on  SaturateOnIntegerOverflow=on  OutDataTypeStr=Inherit: Same as first input
  Cmr1 : Sum  Inputs=-+  InputSameDT=on  SaturateOnIntegerOverflow=on  OutDataTypeStr=Inherit: Same as first input
  Demux : Demux  Outputs=3
  Fcn : Fcn
  Fcn1 : Fcn  Expr=cos(u[1])
  Fid*iq 1 : Product  InputSameDT=on  RndMeth=Zero  SaturateOnIntegerOverflow=on  OutDataTypeStr=Inherit: Same as first input
  Fiq*id1 : Product  InputSameDT=on  RndMeth=Zero  SaturateOnIntegerOverflow=on  OutDataTypeStr=Inherit: Same as first input
  Mux2 : Mux  Inputs=3
  Park : Subsystem
  Parkinv : Subsystem
  dFi/dt=V-Ri...1 : Subsystem
  dthetelec : Gain  Gain=npp  SaturateOnIntegerOverflow=on  OutDataTypeStr=Inherit: Same as input  ParamDataTypeStr=Inherit: Same as input
  idiq : Scope  NumInputPorts=2
  inertie1 : Gain  Gain=1/J  SaturateOnIntegerOverflow=on  OutDataTypeStr=Inherit: Same as input  ParamDataTypeStr=Inherit: Same as input
  thetelec1 : Integrator
  vitesse1 : Integrator
  currents : Outport
  m : Outport  Port=2
  wires:
  Mux2/1 -> currents/1
  Bus Creator2/1 -> m/1
  [Vit] -> Bus Creator2/7  "Vit"
  [Cm] -> Bus Creator2/6  "Cm"
  [ic] -> Bus Creator2/5  "ic"
  [ib] -> Bus Creator2/4  "ib"
  [ia] -> Bus Creator2/3  "ia"
  [Sin] -> Bus Creator2/2  "Sin"
  [Cos] -> Bus Creator2/1  "Cos"
  [ia] -> Mux2/1
  [ib] -> Mux2/2
  [ic] -> Mux2/3
  [thetelec] -> Bus Creator2/8  "thetelec"
  Fcn1/1 -> Parkinv/1(cos), [Cos], Park/1(cos)
  crc/1 -> Cm-Cr1/2
  Park/1(d) -> dFi/dt=V-Ri...1/1(vd)
  dthetelec/1 -> thetelec1/1, dFi/dt=V-Ri...1/6(dthetelec)
  Cmr1/1 -> Cm/1
  Vf/1 -> dFi/dt=V-Ri...1/3(vf)
  Cm/1 -> [Cm], Cm-Cr1/1
  dFi/dt=V-Ri...1/3(Fid) -> Fid*iq 1/1
  dFi/dt=V-Ri...1/2(id) -> idiq/1, Parkinv/3(d), Fiq*id1/2
  Demux/3 -> Park/5(c), [v_cn]
  Demux/1 -> [v_an], Park/3(a)
  Fid*iq 1/1 -> Cmr1/2
  Park/2(q) -> dFi/dt=V-Ri...1/4(vq)
  Parkinv/1(a) -> [ia]
  Fiq*id1/1 -> Cmr1/1
  Fcn/1 -> Parkinv/2(sin), [Sin], Park/2(sin)
  dFi/dt=V-Ri...1/4(iq) -> idiq/2, Parkinv/4(q), Fid*iq 1/2
  dFi/dt=V-Ri...1/1(Fiq) -> Fiq*id1/1
  vitesse1/1 -> [Vit], dthetelec/1
  Demux/2 -> [v_bn], Park/4(b)
  Parkinv/2(b) -> [ib]
  thetelec1/1 -> [thetelec], Fcn/1, Fcn1/1
  Cm-Cr1/1 -> inertie1/1
  inertie1/1 -> vitesse1/1
  Parkinv/3(c) -> [ic]
  voltages/1 -> Demux/1
  [v_an] -> Bus Creator2/9  "v_an"
  [v_bn] -> Bus Creator2/10  "v_bn"
  [v_cn] -> Bus Creator2/11  "v_cn"

== system bibli_SM_QUEVAL_20240121_R2021a/MS bobiné amortisseurs/VOLTAGE MEASUREMENT SYSTEM Converts voltages into  Simulink signals ==
  Mux : Mux  Inputs=3
  v_an : powerlib/Measurements/Voltage Measurement  PhasorSimulation=off  OutputType=Complex  PSBequivalent=0
  v_bn : powerlib/Measurements/Voltage Measurement  PhasorSimulation=off  OutputType=Complex  PSBequivalent=0
  v_cn : powerlib/Measurements/Voltage Measurement  PhasorSimulation=off  OutputType=Complex  PSBequivalent=0
  a : PMIOPort  Side=Left
  b : PMIOPort  Port=2  Side=Left
  c : PMIOPort  Port=3  Side=Left
  n : PMIOPort  Port=4  Side=Left
  voltages : Outport
  wires:
  v_an/1 -> Mux/1
  v_bn/1 -> Mux/2
  Mux/1 -> voltages/1
  v_cn/1 -> Mux/3
  connections:
  v_an/LConn1 -- a/RConn1
  b/RConn1 -- v_bn/LConn1
  c/RConn1 -- v_cn/LConn1
  n/RConn1 -- v_bn/LConn2 -- v_an/LConn2 -- v_cn/LConn2

== system bibli_SM_QUEVAL_20240121_R2021a/PMSM/CURRENT INJECTION SYSTEM Converts Simulink signals into currents ==
  note: in = -ia - ib -ic
      | R=1e6[ohms] is required for simulation with neutral point not grounded
  currents : Inport
  Demux : Demux  Outputs=3
  Snubber a : powerlib/Elements/Series RLC Branch  LConnTagsString=__new0  RConnTagsString=__new0  BranchType=R  Resistance=1e6  Inductance=1e-3  SetiL0=off  InitialCurrent=0  Capacitance=1e-6  Setx0=off  InitialVoltage=0  Measurements=None
  Snubber b : powerlib/Elements/Series RLC Branch  LConnTagsString=__new0  RConnTagsString=__new0  BranchType=R  Resistance=1e6  Inductance=1e-3  SetiL0=off  InitialCurrent=0  Capacitance=1e-6  Setx0=off  InitialVoltage=0  Measurements=None
  Snubber c : powerlib/Elements/Series RLC Branch  LConnTagsString=__new0  RConnTagsString=__new0  BranchType=R  Resistance=1e6  Inductance=1e-3  SetiL0=off  InitialCurrent=0  Capacitance=1e-6  Setx0=off  InitialVoltage=0  Measurements=None
  ia : powerlib/Electrical Sources/Controlled Current Source  Initialize=off  Source_Type=DC  Amplitude=-iao_pd_si  Phase=0  Frequency=0  Measurements=None
  ib : powerlib/Electrical Sources/Controlled Current Source  Initialize=off  Source_Type=DC  Amplitude=-ibo_pd_si  Phase=0  Frequency=0  Measurements=None
  ic : powerlib/Electrical Sources/Controlled Current Source  Initialize=off  Source_Type=DC  Amplitude=-ico_pd_si  Phase=0  Frequency=0  Measurements=None
  a : PMIOPort  Side=Right
  b : PMIOPort  Port=2  Side=Right
  c : PMIOPort  Port=3  Side=Right
  n : PMIOPort  Port=4  Side=Right
  wires:
  Demux/1 -> ia/1
  Demux/2 -> ib/1
  currents/1 -> Demux/1
  Demux/3 -> ic/1
  connections:
  Snubber a/LConn1 -- a/RConn1 -- ia/RConn1
  ib/RConn1 -- Snubber b/LConn1 -- b/RConn1
  Snubber a/RConn1 -- Snubber c/RConn1 -- n/RConn1 -- ic/LConn1 -- Snubber b/RConn1 -- ib/LConn1 -- ia/LConn1
  ic/RConn1 -- c/RConn1 -- Snubber c/LConn1

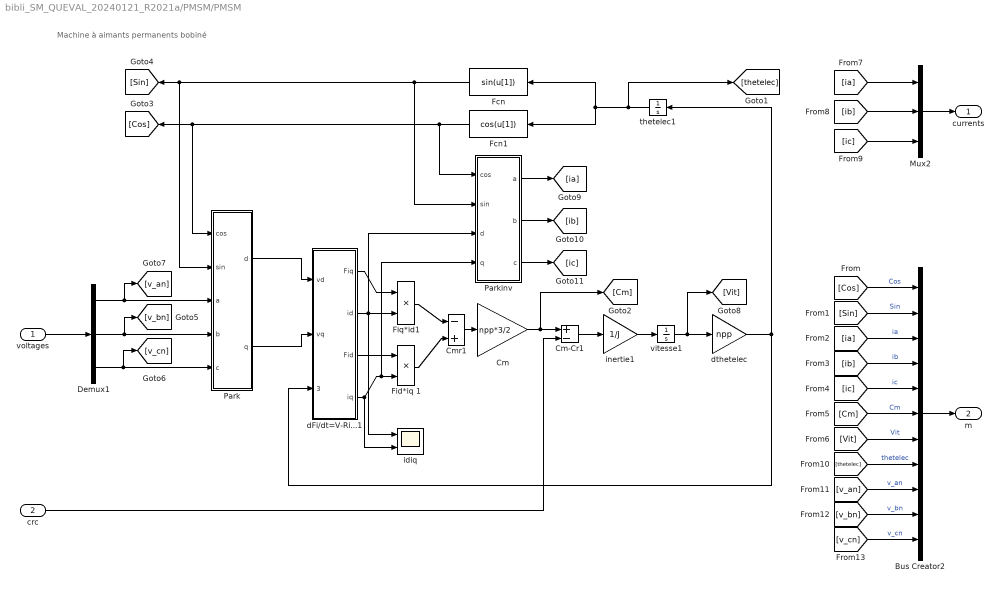
== system bibli_SM_QUEVAL_20240121_R2021a/PMSM/PMSM ==
  note: Machine à aimants permanents bobiné
  voltages : Inport
  crc : Inport  Port=2
  Bus Creator2 : BusCreator  Inputs=11
  Cm : Gain  Gain=npp*3/2  SaturateOnIntegerOverflow=on  OutDataTypeStr=Inherit: Same as input  ParamDataTypeStr=Inherit: Same as input
  Cm-Cr1 : Sum  Inputs=+-  InputSameDT=on  SaturateOnIntegerOverflow=on  OutDataTypeStr=Inherit: Same as first input
  Cmr1 : Sum  Inputs=-+  InputSameDT=on  SaturateOnIntegerOverflow=on  OutDataTypeStr=Inherit: Same as first input
  Demux1 : Demux  Outputs=3
  Fcn : Fcn
  Fcn1 : Fcn  Expr=cos(u[1])
  Fid*iq 1 : Product  InputSameDT=on  SaturateOnIntegerOverflow=on  OutDataTypeStr=Inherit: Same as first input
  Fiq*id1 : Product  InputSameDT=on  SaturateOnIntegerOverflow=on  OutDataTypeStr=Inherit: Same as first input
  Mux2 : Mux  Inputs=3
  Park : Subsystem
  Parkinv : Subsystem
  dFi/dt=V-Ri...1 : Subsystem
  dthetelec : Gain  Gain=npp  SaturateOnIntegerOverflow=on  OutDataTypeStr=Inherit: Same as input  ParamDataTypeStr=Inherit: Same as input
  idiq : Scope  NumInputPorts=2
  inertie1 : Gain  Gain=1/J  SaturateOnIntegerOverflow=on  OutDataTypeStr=Inherit: Same as input  ParamDataTypeStr=Inherit: Same as input
  thetelec1 : Integrator  InitialCondition=pi
  vitesse1 : Integrator
  currents : Outport
  m : Outport  Port=2
  wires:
  Mux2/1 -> currents/1
  Bus Creator2/1 -> m/1
  [Vit] -> Bus Creator2/7  "Vit"
  [Cm] -> Bus Creator2/6  "Cm"
  [ic] -> Bus Creator2/5  "ic"
  [ib] -> Bus Creator2/4  "ib"
  [ia] -> Bus Creator2/3  "ia"
  [Sin] -> Bus Creator2/2  "Sin"
  [Cos] -> Bus Creator2/1  "Cos"
  [ia] -> Mux2/1
  [ib] -> Mux2/2
  [ic] -> Mux2/3
  [thetelec] -> Bus Creator2/8  "thetelec"
  Fiq*id1/1 -> Cmr1/1
  inertie1/1 -> vitesse1/1
  dFi/dt=V-Ri...1/3(Fid) -> Fid*iq 1/1
  Park/1(d) -> dFi/dt=V-Ri...1/1(vd)
  Fid*iq 1/1 -> Cmr1/2
  Park/2(q) -> dFi/dt=V-Ri...1/2(vq)
  Cmr1/1 -> Cm/1
  Demux1/1 -> [v_an], Park/3(a)
  thetelec1/1 -> [thetelec], Fcn/1, Fcn1/1
  vitesse1/1 -> [Vit], dthetelec/1
  Demux1/2 -> [v_bn], Park/4(b)
  Demux1/3 -> [v_cn], Park/5(c)
  Cm/1 -> [Cm], Cm-Cr1/1
  Fcn/1 -> Parkinv/2(sin), [Sin], Park/2(sin)
  Parkinv/1(a) -> [ia]
  Fcn1/1 -> Parkinv/1(cos), [Cos], Park/1(cos)
  dFi/dt=V-Ri...1/2(id) -> idiq/1, Parkinv/3(d), Fiq*id1/2
  Parkinv/2(b) -> [ib]
  dthetelec/1 -> thetelec1/1, dFi/dt=V-Ri...1/3(dthetelec)
  dFi/dt=V-Ri...1/1(Fiq) -> Fiq*id1/1
  Parkinv/3(c) -> [ic]
  dFi/dt=V-Ri...1/4(iq) -> idiq/2, Parkinv/4(q), Fid*iq 1/2
  Cm-Cr1/1 -> inertie1/1
  voltages/1 -> Demux1/1
  crc/1 -> Cm-Cr1/2
  [v_an] -> Bus Creator2/9  "v_an"
  [v_bn] -> Bus Creator2/10  "v_bn"
  [v_cn] -> Bus Creator2/11  "v_cn"

== system bibli_SM_QUEVAL_20240121_R2021a/PMSM/VOLTAGE MEASUREMENT SYSTEM Converts voltages into  Simulink signals ==
  Mux : Mux  Inputs=3
  v_an : powerlib/Measurements/Voltage Measurement  PhasorSimulation=off  OutputType=Complex  PSBequivalent=0
  v_bn : powerlib/Measurements/Voltage Measurement  PhasorSimulation=off  OutputType=Complex  PSBequivalent=0
  v_cn : powerlib/Measurements/Voltage Measurement  PhasorSimulation=off  OutputType=Complex  PSBequivalent=0
  a : PMIOPort  Side=Left
  b : PMIOPort  Port=2  Side=Left
  c : PMIOPort  Port=3  Side=Left
  n : PMIOPort  Port=4  Side=Left
  voltages : Outport
  wires:
  v_an/1 -> Mux/1
  v_bn/1 -> Mux/2
  Mux/1 -> voltages/1
  v_cn/1 -> Mux/3
  connections:
  v_an/LConn1 -- a/RConn1
  b/RConn1 -- v_bn/LConn1
  c/RConn1 -- v_cn/LConn1
  n/RConn1 -- v_bn/LConn2 -- v_an/LConn2 -- v_cn/LConn2

== system bibli_SM_QUEVAL_20240121_R2021a/Park/Clark ==
  a : Inport
  b : Inport  Port=2
  c : Inport  Port=3
  "Clark " : StateSpace  A=[]  B=[]  C=[]  D=K  InitialCondition=0  mask(Matrix Gain){K=Clark}
      mask prompts: K "Gain matrix:"
      mask help: Matrix Gain.
      mask Help: Multiplies input vector by entered matrix to produce output vector (y=Au).
      mask Display: disp('K')
  Demux : Demux  Outputs=3
      settings: DisplayOption=none
  Mux : Mux  Inputs=3
  alpha : Outport  InitialOutput=0  VectorParamsAs1DForOutWhenUnconnected=off
  beta : Outport  Port=2  InitialOutput=0  VectorParamsAs1DForOutWhenUnconnected=off
  o : Outport  Port=3  InitialOutput=0  VectorParamsAs1DForOutWhenUnconnected=off
  wires:
  a/1 -> Mux/1
  b/1 -> Mux/2
  c/1 -> Mux/3
  Mux/1 -> "Clark "/1
  "Clark "/1 -> Demux/1
  Demux/1 -> alpha/1
  Demux/2 -> beta/1
  Demux/3 -> o/1

== system bibli_SM_QUEVAL_20240121_R2021a/Park/Rotation ==
  cos : Inport
  sin : Inport  Port=2
  alpha : Inport  Port=3
  beta : Inport  Port=4
  Product{,1..3} (4 alike) : Product  InputSameDT=on  SaturateOnIntegerOverflow=on  OutDataTypeStr=Inherit: Same as first input
  Sum : Sum  InputSameDT=on  SaturateOnIntegerOverflow=on  OutDataTypeStr=Inherit: Same as first input
  Sum1 : Sum  Inputs=-+  InputSameDT=on  SaturateOnIntegerOverflow=on  OutDataTypeStr=Inherit: Same as first input
  d : Outport  InitialOutput=0  VectorParamsAs1DForOutWhenUnconnected=off
  q : Outport  Port=2  InitialOutput=0  VectorParamsAs1DForOutWhenUnconnected=off
  wires:
  Product/1 -> Sum/1
  Product1/1 -> Sum/2
  sin/1 -> Product1/1, Product2/2
  cos/1 -> Product/1, Product3/1
  Product2/1 -> Sum1/1
  Product3/1 -> Sum1/2
  Sum/1 -> d/1
  Sum1/1 -> q/1
  beta/1 -> Product1/2, Product3/2
  alpha/1 -> Product/2, Product2/1

== system bibli_SM_QUEVAL_20240121_R2021a/Parkinv/ClarkInv ==
  alpha : Inport
  beta : Inport  Port=2
  o : Inport  Port=3
  "ClarkInv " : StateSpace  A=[]  B=[]  C=[]  D=K  InitialCondition=0  mask(Matrix Gain){K=InvClark}
      mask prompts: K "Gain matrix:"
      mask help: Matrix Gain.
      mask Help: Multiplies input vector by entered matrix to produce output vector (y=Au).
      mask Display: disp('K')
  Demux : Demux  Outputs=3
      settings: DisplayOption=none
  Mux : Mux  Inputs=3
  a : Outport  InitialOutput=0  VectorParamsAs1DForOutWhenUnconnected=off
  b : Outport  Port=2  InitialOutput=0  VectorParamsAs1DForOutWhenUnconnected=off
  c : Outport  Port=3  InitialOutput=0  VectorParamsAs1DForOutWhenUnconnected=off
  wires:
  alpha/1 -> Mux/1
  beta/1 -> Mux/2
  o/1 -> Mux/3
  Mux/1 -> "ClarkInv "/1
  "ClarkInv "/1 -> Demux/1
  Demux/1 -> a/1
  Demux/2 -> b/1
  Demux/3 -> c/1

== system bibli_SM_QUEVAL_20240121_R2021a/Parkinv/Rotation Inverse ==
  cos : Inport
  sin : Inport  Port=2
  d : Inport  Port=3
  q : Inport  Port=4
  Product{,1..3} (4 alike) : Product  InputSameDT=on  SaturateOnIntegerOverflow=on  OutDataTypeStr=Inherit: Same as first input
  Sum : Sum  Inputs=+-  InputSameDT=on  SaturateOnIntegerOverflow=on  OutDataTypeStr=Inherit: Same as first input
  Sum1 : Sum  InputSameDT=on  SaturateOnIntegerOverflow=on  OutDataTypeStr=Inherit: Same as first input
  alpha : Outport  InitialOutput=0  VectorParamsAs1DForOutWhenUnconnected=off
  beta : Outport  Port=2  InitialOutput=0  VectorParamsAs1DForOutWhenUnconnected=off
  wires:
  Product/1 -> Sum/1
  Product1/1 -> Sum/2
  sin/1 -> Product1/1, Product2/2
  cos/1 -> Product/1, Product3/1
  Product2/1 -> Sum1/1
  Product3/1 -> Sum1/2
  Sum/1 -> alpha/1
  Sum1/1 -> beta/1
  q/1 -> Product1/2, Product3/2
  d/1 -> Product/2, Product2/1

== system bibli_SM_QUEVAL_20240121_R2021a/MS bobiné/MS bobiné/Park1 ==
  cos : Inport
  sin : Inport  Port=2
  a : Inport  Port=3
  b : Inport  Port=4
  c : Inport  Port=5
  Clark : Subsystem
  Rotation : Subsystem
  d : Outport  InitialOutput=0  VectorParamsAs1DForOutWhenUnconnected=off
  q : Outport  Port=2  InitialOutput=0  VectorParamsAs1DForOutWhenUnconnected=off
  wires:
  Clark/2(beta) -> Rotation/4(beta)
  Clark/1(alpha) -> Rotation/3(alpha)
  a/1 -> Clark/1(a)
  sin/1 -> Rotation/2(sin)
  c/1 -> Clark/3(c)
  b/1 -> Clark/2(b)
  Rotation/2(q) -> q/1
  Rotation/1(d) -> d/1
  cos/1 -> Rotation/1(cos)

== system bibli_SM_QUEVAL_20240121_R2021a/MS bobiné/MS bobiné/Parkinv1 ==
  cos : Inport
  sin : Inport  Port=2
  d : Inport  Port=3
  q : Inport  Port=4
  ClarkInv : Subsystem
  Rotation Inverse : Subsystem
  a : Outport  InitialOutput=0  VectorParamsAs1DForOutWhenUnconnected=off
  b : Outport  Port=2  InitialOutput=0  VectorParamsAs1DForOutWhenUnconnected=off
  c : Outport  Port=3  InitialOutput=0  VectorParamsAs1DForOutWhenUnconnected=off
  wires:
  Rotation Inverse/2(beta) -> ClarkInv/2(beta)
  q/1 -> Rotation Inverse/4(q)
  ClarkInv/3(c) -> c/1
  d/1 -> Rotation Inverse/3(d)
  ClarkInv/2(b) -> b/1
  sin/1 -> Rotation Inverse/2(sin)
  ClarkInv/1(a) -> a/1
  cos/1 -> Rotation Inverse/1(cos)
  Rotation Inverse/1(alpha) -> ClarkInv/1(alpha)

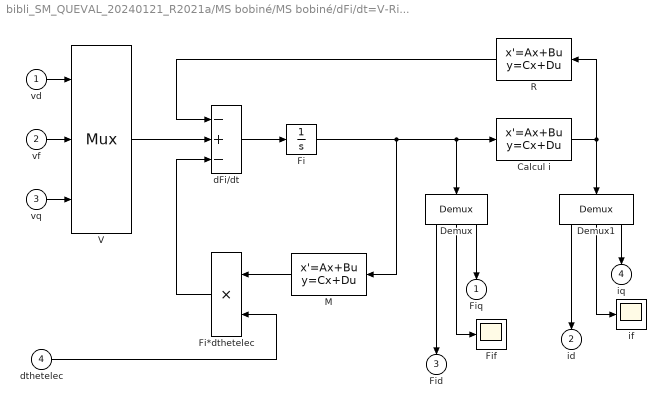
== system bibli_SM_QUEVAL_20240121_R2021a/MS bobiné/MS bobiné/dFi/dt=V-Ri... ==
  vd : Inport
  vf : Inport  Port=2
  vq : Inport  Port=3
  dthetelec : Inport  Port=4
  Calcul i : StateSpace  A=[]  B=[]  C=[]  D=K  InitialCondition=0  mask(Matrix gain){K=INVL}
      mask prompts: K "Gain matrix:"
      mask help: Matrix Gain.
      mask Help: Multiplies input vector by entered matrix to produce output vector (y=Au).
      mask Display: disp('Matrice')
  Demux : Demux  Outputs=3
      settings: DisplayOption=none
  Demux1 : Demux  Outputs=3
      settings: DisplayOption=none
  Fi : Integrator  InitialCondition=[0 0 0]
  Fi*dthetelec : Product  InputSameDT=on  RndMeth=Zero  SaturateOnIntegerOverflow=on  OutDataTypeStr=Inherit: Same as first input
  Fif : Scope
  M : StateSpace  A=[]  B=[]  C=[]  D=K  InitialCondition=0  mask(Matrix gain){K=M}
      mask prompts: K "Gain matrix:"
      mask help: Matrix Gain.
      mask Help: Multiplies input vector by entered matrix to produce output vector (y=Au).
      mask Display: disp('Matrice')
  R : StateSpace  A=[]  B=[]  C=[]  D=K  InitialCondition=0  mask(Matrix gain){K=R}
      mask prompts: K "Gain matrix:"
      mask help: Matrix Gain.
      mask Help: Multiplies input vector by entered matrix to produce output vector (y=Au).
      mask Display: disp('Matrice')
  V : Mux  Inputs=3
  dFi/dt : Sum  Inputs=-+-  InputSameDT=on  SaturateOnIntegerOverflow=on  OutDataTypeStr=Inherit: Same as first input
  if : Scope
  Fiq : Outport  InitialOutput=0  VectorParamsAs1DForOutWhenUnconnected=off
  id : Outport  Port=2  InitialOutput=0  VectorParamsAs1DForOutWhenUnconnected=off
  Fid : Outport  Port=3  InitialOutput=0  VectorParamsAs1DForOutWhenUnconnected=off
  iq : Outport  Port=4  InitialOutput=0  VectorParamsAs1DForOutWhenUnconnected=off
  wires:
  Demux1/2 -> if/1
  Demux1/3 -> iq/1
  Demux/2 -> Fif/1
  Demux/3 -> Fiq/1
  Demux1/1 -> id/1
  vq/1 -> V/3
  vf/1 -> V/2
  Fi*dthetelec/1 -> dFi/dt/3
  M/1 -> Fi*dthetelec/1
  Demux/1 -> Fid/1
  vd/1 -> V/1
  dFi/dt/1 -> Fi/1
  R/1 -> dFi/dt/1
  V/1 -> dFi/dt/2
  Calcul i/1 -> Demux1/1, R/1
  dthetelec/1 -> Fi*dthetelec/2
  Fi/1 -> M/1, Demux/1, Calcul i/1

== system bibli_SM_QUEVAL_20240121_R2021a/MS bobiné amortisseurs/MS bobiné amortisseurs/Park ==
  cos : Inport
  sin : Inport  Port=2
  a : Inport  Port=3
  b : Inport  Port=4
  c : Inport  Port=5
  Clark : Subsystem
  Rotation : Subsystem
  d : Outport  InitialOutput=0  VectorParamsAs1DForOutWhenUnconnected=off
  q : Outport  Port=2  InitialOutput=0  VectorParamsAs1DForOutWhenUnconnected=off
  wires:
  Clark/2(beta) -> Rotation/4(beta)
  Clark/1(alpha) -> Rotation/3(alpha)
  a/1 -> Clark/1(a)
  sin/1 -> Rotation/2(sin)
  c/1 -> Clark/3(c)
  b/1 -> Clark/2(b)
  Rotation/2(q) -> q/1
  Rotation/1(d) -> d/1
  cos/1 -> Rotation/1(cos)

== system bibli_SM_QUEVAL_20240121_R2021a/MS bobiné amortisseurs/MS bobiné amortisseurs/Parkinv ==
  cos : Inport
  sin : Inport  Port=2
  d : Inport  Port=3
  q : Inport  Port=4
  ClarkInv : Subsystem
  Rotation Inverse : Subsystem
  a : Outport  InitialOutput=0  VectorParamsAs1DForOutWhenUnconnected=off
  b : Outport  Port=2  InitialOutput=0  VectorParamsAs1DForOutWhenUnconnected=off
  c : Outport  Port=3  InitialOutput=0  VectorParamsAs1DForOutWhenUnconnected=off
  wires:
  Rotation Inverse/2(beta) -> ClarkInv/2(beta)
  q/1 -> Rotation Inverse/4(q)
  ClarkInv/3(c) -> c/1
  d/1 -> Rotation Inverse/3(d)
  ClarkInv/2(b) -> b/1
  sin/1 -> Rotation Inverse/2(sin)
  ClarkInv/1(a) -> a/1
  cos/1 -> Rotation Inverse/1(cos)
  Rotation Inverse/1(alpha) -> ClarkInv/1(alpha)

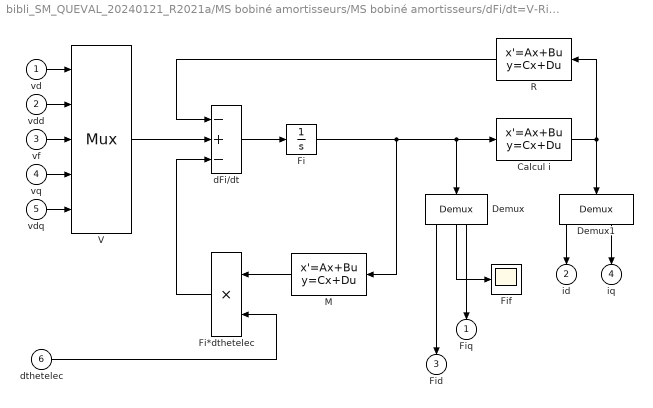
== system bibli_SM_QUEVAL_20240121_R2021a/MS bobiné amortisseurs/MS bobiné amortisseurs/dFi/dt=V-Ri...1 ==
  vd : Inport
  vdd : Inport  Port=2
  vf : Inport  Port=3
  vq : Inport  Port=4
  vdq : Inport  Port=5
  dthetelec : Inport  Port=6
  Calcul i : StateSpace  A=[]  B=[]  C=[]  D=K  InitialCondition=0  mask(Matrix gain){K=INVL}
      mask prompts: K "Gain matrix:"
      mask help: Matrix Gain.
      mask Help: Multiplies input vector by entered matrix to produce output vector (y=Au).
      mask Display: disp('Matrice')
  Demux : Demux  Outputs=5
      settings: DisplayOption=none
  Demux1 : Demux  Outputs=5
      settings: DisplayOption=none
  Fi : Integrator  InitialCondition=[0 0 0 0 0]
  Fi*dthetelec : Product  InputSameDT=on  RndMeth=Zero  SaturateOnIntegerOverflow=on  OutDataTypeStr=Inherit: Same as first input
  Fif : Scope
  M : StateSpace  A=[]  B=[]  C=[]  D=K  InitialCondition=0  mask(Matrix gain){K=M}
      mask prompts: K "Gain matrix:"
      mask help: Matrix Gain.
      mask Help: Multiplies input vector by entered matrix to produce output vector (y=Au).
      mask Display: disp('Matrice')
  R : StateSpace  A=[]  B=[]  C=[]  D=K  InitialCondition=0  mask(Matrix gain){K=R}
      mask prompts: K "Gain matrix:"
      mask help: Matrix Gain.
      mask Help: Multiplies input vector by entered matrix to produce output vector (y=Au).
      mask Display: disp('Matrice')
  V : Mux  Inputs=5
  dFi/dt : Sum  Inputs=-+-  InputSameDT=on  SaturateOnIntegerOverflow=on  OutDataTypeStr=Inherit: Same as first input
  Fiq : Outport  InitialOutput=0  VectorParamsAs1DForOutWhenUnconnected=off
  id : Outport  Port=2  InitialOutput=0  VectorParamsAs1DForOutWhenUnconnected=off
  Fid : Outport  Port=3  InitialOutput=0  VectorParamsAs1DForOutWhenUnconnected=off
  iq : Outport  Port=4  InitialOutput=0  VectorParamsAs1DForOutWhenUnconnected=off
  wires:
  Demux/3 -> Fif/1
  Fi*dthetelec/1 -> dFi/dt/3
  M/1 -> Fi*dthetelec/1
  Demux/1 -> Fid/1
  Demux/4 -> Fiq/1
  Demux1/1 -> id/1
  Demux1/4 -> iq/1
  vdq/1 -> V/5
  vq/1 -> V/4
  vf/1 -> V/3
  vdd/1 -> V/2
  vd/1 -> V/1
  dFi/dt/1 -> Fi/1
  R/1 -> dFi/dt/1
  V/1 -> dFi/dt/2
  Calcul i/1 -> Demux1/1, R/1
  dthetelec/1 -> Fi*dthetelec/2
  Fi/1 -> M/1, Demux/1, Calcul i/1

== system bibli_SM_QUEVAL_20240121_R2021a/PMSM/PMSM/Park ==
  cos : Inport
  sin : Inport  Port=2
  a : Inport  Port=3
  b : Inport  Port=4
  c : Inport  Port=5
  Clark : Subsystem
  Rotation : Subsystem
  d : Outport  InitialOutput=0  VectorParamsAs1DForOutWhenUnconnected=off
  q : Outport  Port=2  InitialOutput=0  VectorParamsAs1DForOutWhenUnconnected=off
  wires:
  Clark/2(beta) -> Rotation/4(beta)
  Clark/1(alpha) -> Rotation/3(alpha)
  a/1 -> Clark/1(a)
  sin/1 -> Rotation/2(sin)
  c/1 -> Clark/3(c)
  b/1 -> Clark/2(b)
  Rotation/2(q) -> q/1
  Rotation/1(d) -> d/1
  cos/1 -> Rotation/1(cos)

== system bibli_SM_QUEVAL_20240121_R2021a/PMSM/PMSM/Parkinv ==
  cos : Inport
  sin : Inport  Port=2
  d : Inport  Port=3
  q : Inport  Port=4
  ClarkInv : Subsystem
  Rotation Inverse : Subsystem
  a : Outport  InitialOutput=0  VectorParamsAs1DForOutWhenUnconnected=off
  b : Outport  Port=2  InitialOutput=0  VectorParamsAs1DForOutWhenUnconnected=off
  c : Outport  Port=3  InitialOutput=0  VectorParamsAs1DForOutWhenUnconnected=off
  wires:
  Rotation Inverse/2(beta) -> ClarkInv/2(beta)
  q/1 -> Rotation Inverse/4(q)
  ClarkInv/3(c) -> c/1
  d/1 -> Rotation Inverse/3(d)
  ClarkInv/2(b) -> b/1
  sin/1 -> Rotation Inverse/2(sin)
  ClarkInv/1(a) -> a/1
  cos/1 -> Rotation Inverse/1(cos)
  Rotation Inverse/1(alpha) -> ClarkInv/1(alpha)

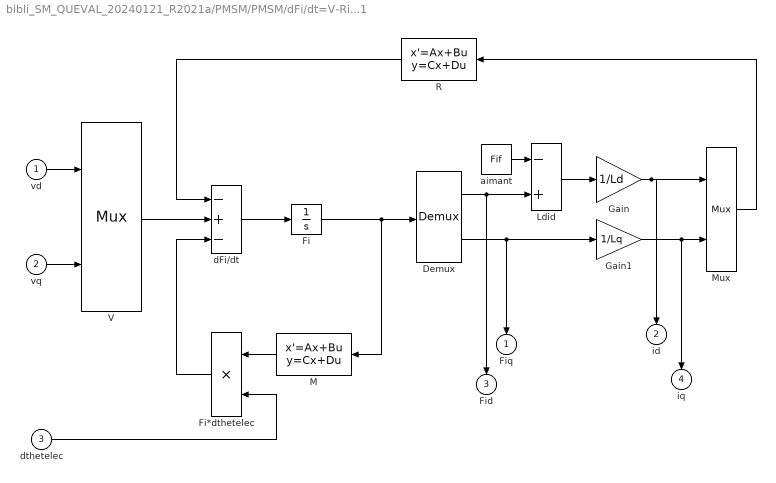
== system bibli_SM_QUEVAL_20240121_R2021a/PMSM/PMSM/dFi/dt=V-Ri...1 ==
  vd : Inport
  vq : Inport  Port=2
  dthetelec : Inport  Port=3
  Demux : Demux  Outputs=2
      settings: DisplayOption=none
  Fi : Integrator  InitialCondition=[Fif 0]
  Fi*dthetelec : Product  InputSameDT=on  SaturateOnIntegerOverflow=on  OutDataTypeStr=Inherit: Same as first input
  Gain : Gain  Gain=1/Ld  SaturateOnIntegerOverflow=on  OutDataTypeStr=Inherit: Same as input  ParamDataTypeStr=Inherit: Same as input
  Gain1 : Gain  Gain=1/Lq  SaturateOnIntegerOverflow=on  OutDataTypeStr=Inherit: Same as input  ParamDataTypeStr=Inherit: Same as input
  Ldid : Sum  Inputs=-+  InputSameDT=on  SaturateOnIntegerOverflow=on  OutDataTypeStr=Inherit: Same as first input
  M : StateSpace  A=[]  B=[]  C=[]  D=K  InitialCondition=0  mask(Matrix gain){K=M}
      mask prompts: K "Gain matrix:"
      mask help: Matrix Gain.
      mask Help: Multiplies input vector by entered matrix to produce output vector (y=Au).
      mask Display: disp('Matrice')
  Mux : Mux  Inputs=2
  R : StateSpace  A=[]  B=[]  C=[]  D=K  InitialCondition=0  mask(Matrix gain){K=R}
      mask prompts: K "Gain matrix:"
      mask help: Matrix Gain.
      mask Help: Multiplies input vector by entered matrix to produce output vector (y=Au).
      mask Display: disp('Matrice')
  V : Mux  Inputs=2
  aimant : Constant  Value=Fif
  dFi/dt : Sum  Inputs=-+-  InputSameDT=on  SaturateOnIntegerOverflow=on  OutDataTypeStr=Inherit: Same as first input
  Fiq : Outport  InitialOutput=0  VectorParamsAs1DForOutWhenUnconnected=off
  id : Outport  Port=2  InitialOutput=0  VectorParamsAs1DForOutWhenUnconnected=off
  Fid : Outport  Port=3  InitialOutput=0  VectorParamsAs1DForOutWhenUnconnected=off
  iq : Outport  Port=4  InitialOutput=0  VectorParamsAs1DForOutWhenUnconnected=off
  wires:
  Mux/1 -> R/1
  Gain1/1 -> iq/1, Mux/2
  Gain/1 -> id/1, Mux/1
  Demux/2 -> Fiq/1, Gain1/1
  Ldid/1 -> Gain/1
  aimant/1 -> Ldid/1
  Demux/1 -> Fid/1, Ldid/2
  Fi*dthetelec/1 -> dFi/dt/3
  M/1 -> Fi*dthetelec/1
  vq/1 -> V/2
  vd/1 -> V/1
  dFi/dt/1 -> Fi/1
  R/1 -> dFi/dt/1
  V/1 -> dFi/dt/2
  dthetelec/1 -> Fi*dthetelec/2
  Fi/1 -> Demux/1, M/1

== system bibli_SM_QUEVAL_20240121_R2021a/MS bobiné/MS bobiné/Park1/Clark ==
  a : Inport
  b : Inport  Port=2
  c : Inport  Port=3
  "Clark " : StateSpace  A=[]  B=[]  C=[]  D=K  InitialCondition=0  mask(Matrix Gain){K=Clark}
      mask prompts: K "Gain matrix:"
      mask help: Matrix Gain.
      mask Help: Multiplies input vector by entered matrix to produce output vector (y=Au).
      mask Display: disp('K')
  Demux : Demux  Outputs=3
      settings: DisplayOption=none
  Mux : Mux  Inputs=3
  alpha : Outport  InitialOutput=0  VectorParamsAs1DForOutWhenUnconnected=off
  beta : Outport  Port=2  InitialOutput=0  VectorParamsAs1DForOutWhenUnconnected=off
  o : Outport  Port=3  InitialOutput=0  VectorParamsAs1DForOutWhenUnconnected=off
  wires:
  Demux/3 -> o/1
  Demux/2 -> beta/1
  Demux/1 -> alpha/1
  "Clark "/1 -> Demux/1
  Mux/1 -> "Clark "/1
  c/1 -> Mux/3
  b/1 -> Mux/2
  a/1 -> Mux/1
